simulink model "inverse_control"  (R2020a)
settings: Solver=VariableStepAuto  StartTime=0.0  StopTime=700  RelTol=1e-3
libraries: simulink x2
settings Model: Creator=elkin  LastModifiedBy=elkin

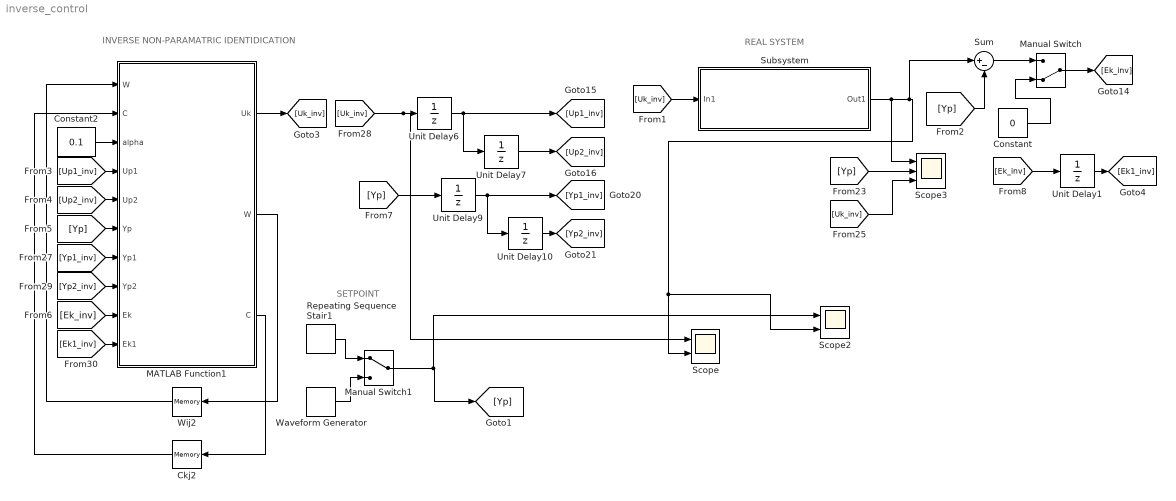
== system inverse_control ==
  note: SETPOINT
  note: REAL SYSTEM
  note: INVERSE NON-PARAMATRIC IDENTIDICATION
  Ckj2 : Memory  InitialCondition=[0.839221357445656,-0.492336931902849,-0.0237000817730927,0.423645174386349,0.332773233415874,0.343451601382383,0.300843854457738,-0.345695860840541,-1.38941797440746,1.97385835508798]
  Constant : Constant  Value=0
  Constant2 : Constant  Value=0.1
  MATLAB Function1 : MATLAB Function  TreatAsAtomicUnit=on
  Manual Switch : ManualSwitch  CurrentSetting=0
  Manual Switch1 : ManualSwitch
  Repeating Sequence Stair1 : simulink/Sources/Repeating Sequence Stair  OutValues=[0 0.2 0 0.4 0.8 0.4 1].'  tsamp=15  OutMin=[]  OutMax=[]  OutDataTypeStr=double  OutputDataTypeScalingMode=double  OutDataType=fixdt(0,8)  ConRadixGroup=Best Precision: Vector-wise  OutScaling=2^-12
  Scope : Scope  NumInputPorts=2
  Scope2 : Scope  NumInputPorts=2
  Scope3 : Scope  NumInputPorts=3
  Subsystem : Subsystem
  Sum : Sum  Inputs=|+-
  Unit Delay{1,6..7,9..10} (5 alike) : UnitDelay  SampleTime=-1  HasFrameUpgradeWarning=on
  Waveform Generator : simulink/Sources/Waveform Generator  OutMin=[]  OutMax=[]  OutDataTypeStr=double  SelectedSignal=1  Signals=sin(1, 0.03, 0)  BlockNames=MultiportSwitch_45ff84b921fe4c9  SampleTime=0.1
  Wij2 : Memory  InitialCondition=[1.49930493018781,-0.503694725931312,0.0830359125805244,0.796730196483625,0.0925003620229678,-1.12296438657777;1.24511313974662,-1.60991886897643,1.06070835587408,-0.353954943215072,1.75938068882501,-1.46592515473037;0.774897668736740,0.619330356200666,-0.298758171776083,-0.549111358464897,0.304171327425112,0.342508257913762;-0.649561231954874,-0.0955935085572402,1.45396012318110,-0.112171490344236,2.00515410025399,1.35675666336286;0.277748241795899,0.722729967047914,0.442567808872045,-1.12843010471380,-0.753840114719591,-0.402302730288129;-0.665764601113419,0.150902269481346,1.10147671867647,-0.562421555627248,0.460475015963419,0.643589225798979;-0.498173456629167,0.396521492155548,0.0340892547359703,-0.274581606969944,-0.355008257310871,0.497819065807182;-0.692454593367076,-1.53411961753938,-0.743965182737245,-0.0435969043919127,0.508371096137286,-0.956713878805398;-0.889034173119795,-1.04458976037129,-1.57326079550751,-0.158494158363639,0.496030124046587,0.00853902383160640;-0.706331617454330,-0.731947309195436,0.473265797489702,0.932504671355998,-1.86103178211945,-0.0384540201041527]
  wires:
  Unit Delay7/1 -> [Up2_inv]
  Unit Delay6/1 -> [Up1_inv], Unit Delay7/1
  [Uk_inv] -> Scope/1, Unit Delay6/1
  Subsystem/1(Out1) -> Scope3/1, Sum/1, Scope2/2, Scope/2
  Constant/1 -> Manual Switch/2
  [Uk_inv] -> Scope3/3
  [Yp1_inv] -> MATLAB Function1/7(Yp1)
  MATLAB Function1/2(W) -> Wij2/1
  [Yp2_inv] -> MATLAB Function1/8(Yp2)
  Wij2/1 -> MATLAB Function1/1("W ")
  MATLAB Function1/3(C) -> Ckj2/1
  [Ek_inv] -> MATLAB Function1/9(Ek)
  [Up1_inv] -> MATLAB Function1/4(Up1)
  [Up2_inv] -> MATLAB Function1/5(Up2)
  [Yp] -> MATLAB Function1/6(Yp)
  Constant2/1 -> MATLAB Function1/3(alpha)
  Ckj2/1 -> MATLAB Function1/2("C ")
  [Ek1_inv] -> MATLAB Function1/10(Ek1)
  MATLAB Function1/1(Uk) -> [Uk_inv]
  [Yp] -> Unit Delay9/1
  Unit Delay9/1 -> [Yp1_inv], Unit Delay10/1
  Unit Delay10/1 -> [Yp2_inv]
  Unit Delay1/1 -> [Ek1_inv]
  [Ek_inv] -> Unit Delay1/1
  [Yp] -> Scope3/2
  [Uk_inv] -> Subsystem/1(In1)
  Repeating Sequence Stair1/1 -> Manual Switch1/1
  Waveform Generator/1 -> Manual Switch1/2
  Manual Switch1/1 -> Scope2/1, [Yp]
  [Yp] -> Sum/2
  Sum/1 -> Manual Switch/1
  Manual Switch/1 -> [Ek_inv]

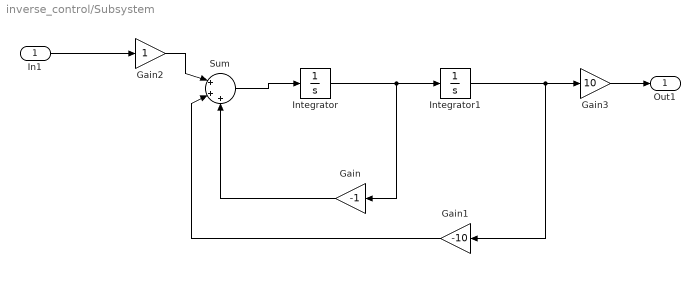
== system inverse_control/Subsystem ==
  In1 : Inport
  Gain : Gain  Gain=-1
  Gain1 : Gain  Gain=-10
  Gain2 : Gain
  Gain3 : Gain  Gain=10
  Integrator : Integrator
  Integrator1 : Integrator
  Sum : Sum  Inputs=|+++
  Out1 : Outport  VectorParamsAs1DForOutWhenUnconnected=off
  wires:
  Integrator/1 -> Gain/1, Integrator1/1
  Gain2/1 -> Sum/1
  Gain1/1 -> Sum/2
  Sum/1 -> Integrator/1
  Integrator1/1 -> Gain3/1, Gain1/1
  Gain/1 -> Sum/3
  In1/1 -> Gain2/1
  Gain3/1 -> Out1/1

== matlab function inverse_control/MATLAB Function1 ==
  data: W input; Uk output; C input; alpha input; Up1 input; Up2 input; Yp input; Yp1 input; Yp2 input; Ek input; W output; C output; Ek1 input
function [Uk, W, C] = fcn(W, C, alpha, Up1, Up2, Yp, Yp1, Yp2, Ek, Ek1)
    % Define input vector
    X = [Up1 Up2 Yp Yp1 Yp2 Ek1];
    
    % Calculate Aj in the hidden layer
    Aj = W*X';
    
    % Activation function of the hidden layer
    H = tanh(Aj);
    
    % Calculate Ak in the output layer
    Ak = C'*H;
    
    % Activation function of the output layer
    Uk = Ak;
    
    % Update C matrix
    C = C + alpha*Ek*H;
    
    % Update W matrix
    Hd = sech(Aj).^2;
    W = W + alpha*Ek*(C.*Hd)*X;
